simulink subsystem "ForwardKinematicsRAD"  (R2024b)
settings: Solver=VariableStepAuto  StartTime=0.0  StopTime=10.0  RelTol=1e-3
undefined symbols (not defined in the file or in its folder): l, r
settings Model: Creator=Matthew  LastModifiedBy=Matthew

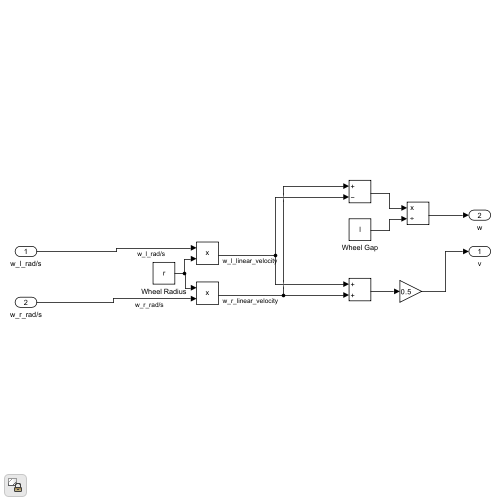
[thumbnail: Simulink's stored preview of the top-level diagram]
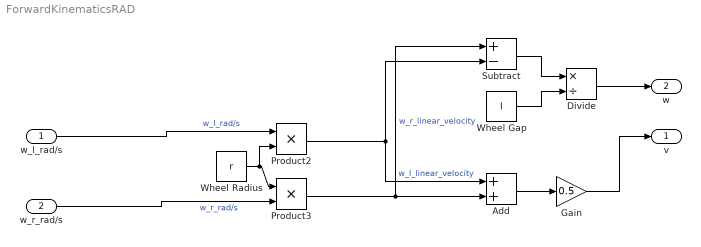
== system ForwardKinematicsRAD ==
  w_l_rad/s : Inport
  w_r_rad/s : Inport  Port=2
  Add : Sum
  Divide : Product  Inputs=*/  SaturateOnIntegerOverflow=on
  Gain : Gain  Gain=0.5
  Product2 : Product
  Product3 : Product
  Subtract : Sum  Inputs=+-
  Wheel Gap : Constant  Value=l
  Wheel Radius : Constant  Value=r
  v : Outport
  w : Outport  Port=2
  wires:
  w_l_rad/s/1 -> Product2/1  "w_l_rad/s"
  w_r_rad/s/1 -> Product3/2  "w_r_rad/s"
  Wheel Radius/1 -> Product2/2, Product3/1
  Product2/1 -> Subtract/2, Add/1  "w_l_linear_velocity"
  Product3/1 -> Add/2, Subtract/1  "w_r_linear_velocity"
  Add/1 -> Gain/1
  Gain/1 -> v/1
  Subtract/1 -> Divide/1
  Wheel Gap/1 -> Divide/2
  Divide/1 -> w/1
